simulink model "ClutchControl"  (R2020b)
settings: Solver=VariableStepAuto  StartTime=0.0  StopTime=5  RelTol=1e-3
values from neighbouring files (symbols this model uses):
  A = [0 -1 r; 2*k/m 0 0;-2*k*r/J -Km*k1*k2/J/R -b/J]    [Ex_uncertainties2018_1.m]    (also in Lab_Clutch.m = [0 1 0 0; -k/Jl -Bl/Jl k/Jl 0; 0 0 0 1; k/Jm 0 -k/Jm -Bm/Jm]; halfLinearModel.m = [0 1 0 0 0 0 0 0)
  B = [0;0;-1/J]    [Ex_uncertainties2018_1.m]    (also in Lab_Clutch.m = [0; 0; 0; 1/Jm]; halfLinearModel.m = [0 0 0 0 0 0)
  C = [0 1 0]    [Ex_uncertainties2018_1.m]    (also in Lab_Clutch.m = [1 0 0 0]; halfLinearModel.m = [A(6,:))
  D = 0    [Ex_uncertainties2018_1.m]    (also in Lab_Clutch.m; halfLinearModel.m = [B(6,:))
undefined symbols (not defined in the file or in its folder): khinf
libraries: pid_lib x1
settings Model: Creator=DELL  LastModifiedBy=DELL

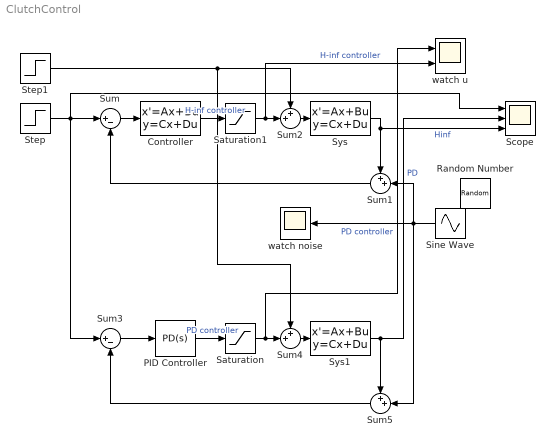
== system ClutchControl ==
  Controller : StateSpace  A=khinf.A  B=khinf.B  C=khinf.C  D=khinf.D  InitialCondition=0
  PID Controller : pid_lib/PID Controller  Controller=PD  Form=Parallel  TimeDomain=Continuous-time  UseExternalTs=off  SampleTime=-1  IntegratorMethod=Forward Euler  FilterMethod=Forward Euler  ControllerParametersSource=internal  P=0.3  I=1  D=0.0033  UseFilter=on  N=100000  TunerSelectOption=Transfer Function Based (PID Tuner App)  InitialConditionSource=internal  InitialConditionForIntegrator=0  InitialConditionForFilter=0  DifferentiatorICPrevScaledInput=0  ExternalReset=none  TrackingMode=off  Kt=1  LimitOutput=off  SatLimitsSource=internal  UpperSaturationLimit=inf  LowerSaturationLimit=-inf  LinearizeAsGain=on  AntiWindupMode=none  Kb=1  POutMin=[]  POutMax=[]  IOutMin=[]  IOutMax=[]  DOutMin=[]  DOutMax=[]  NOutMin=[]  NOutMax=[]  SumOutMin=[]  SumOutMax=[]  SaturationOutMin=[]  SaturationOutMax=[]  PParamMin=[]  PParamMax=[]  IParamMin=[]  IParamMax=[]  DParamMin=[]  DParamMax=[]  NParamMin=[]  NParamMax=[]  KbParamMin=[]  KbParamMax=[]  KtParamMin=[]  KtParamMax=[]  KbOutMin=[]  KbOutMax=[]  KtOutMin=[]  KtOutMax=[]  IntegratorOutMin=[]  IntegratorOutMax=[]  FilterOutMin=[]  FilterOutMax=[]  SumI1OutMin=[]  SumI1OutMax=[]  SumI2OutMin=[]  SumI2OutMax=[]  SumI3OutMin=[]  SumI3OutMax=[]  SumI4OutMin=[]  SumI4OutMax=[]  SumDOutMin=[]  SumDOutMax=[]  DifferentiatorOutMin=[]  DifferentiatorOutMax=[]  FilterDiffOutCoefMin=[]  FilterDiffOutCoefMax=[]  ReciprocalOutMin=[]  ReciprocalOutMax=[]  SumDenOutMin=[]  SumDenOutMax=[]  SumNumOutMin=[]  SumNumOutMax=[]  DivideOutMin=[]  DivideOutMax=[]  UdiffTsProdOutMin=[]  UdiffTsProdOutMax=[]  NTsProdOutMin=[]  NTsProdOutMax=[]  UintegralTsProdOutMin=[]  UintegralTsProdOutMax=[]  UngainTsProdOutMin=[]  UngainTsProdOutMax=[]  IntegratorContinuousStateAttributes=''  IntegratorStateMustResolveToSignalObject=off  IntegratorRTWStateStorageClass=Auto  FilterContinuousStateAttributes=''  FilterStateMustResolveToSignalObject=off  FilterRTWStateStorageClass=Auto  ParallelPVariant=InternalParameters  IdealPVariant=Disabled  IVariant=Disabled  DVariant=InternalParameters  IntegratorVariant=Disabled  SatVariant=Disabled  AWVariant=Disabled  PCopyVariant=Disabled  TRVariant=Disabled  FdbkBlocksVariant=Forward  IdealPFdbkVariant=Disabled  SatFdbkVariant=Disabled  DerivativeFilterVariant=ContFilter  NVariant=InternalParameters  NCopyVariant=Disabled  FilterICVariant=InternalICsFilter  IntegratorICVariant=Disabled  ExternalResetVariant=Disabled  TRSumVariant=Passthrough  SumFdbkVariant=Disabled  SumVariant=Sum_PD  TsampFilterVariant=InternalTs  TsampNgainVariant=Passthrough  TsampIntegralVariant=Disabled_SignalSpec  ExternalSaturationOutDataTypeStr=Inherit: Same as second input
  Random Number : RandomNumber  Variance=0.0001  SampleTime=0.1
  Saturation : Saturate  UpperLimit=1  LowerLimit=-1
  Saturation1 : Saturate  UpperLimit=1  LowerLimit=-1
  Scope : Scope  NumInputPorts=3
  Sine Wave : Sin  Amplitude=0.1  Frequency=800  SampleTime=0
  Step : Step  SampleTime=0
  Step1 : Step  Time=3  After=0.1  SampleTime=0
  Sum : Sum  Inputs=|+-
  Sum{1..2,4..5} (4 alike) : Sum  Inputs=++|
  Sum3 : Sum  Inputs=|+-
  Sys : StateSpace  A=A  B=B  C=C  D=D  InitialCondition=0
  Sys1 : StateSpace  A=A  B=B  C=C  D=D  InitialCondition=0
  watch noise : Scope
  watch u : Scope  NumInputPorts=2
  wires:
  Sys/1 -> Scope/3, Sum1/1  "Hinf"
  Sum1/1 -> Sum/2
  Controller/1 -> Saturation1/1  "H-inf controller"
  Sum/1 -> Controller/1
  Sum2/1 -> Sys/1
  Sine Wave/1 -> Sum5/2, watch noise/1, Sum1/2
  Step/1 -> Scope/1, Sum3/1, Sum/1
  Step1/1 -> Sum2/1, Sum4/1
  PID Controller/1 -> Saturation/1  "PD controller"
  Sys1/1 -> Scope/2, Sum5/1  "PD"
  Sum5/1 -> Sum3/2
  Sum4/1 -> Sys1/1
  Sum3/1 -> PID Controller/1
  Saturation1/1 -> watch u/2, Sum2/2  "H-inf controller"
  Saturation/1 -> watch u/1, Sum4/2  "PD controller"
